simulink model "Ext_Springs_CS9"  (Simulink 8.8)
settings: Solver=ode45  StartTime=0  StopTime=10  FixedStep=0.001  RelTol=1e-3  AbsTol=1e-6
PreLoadFcn:
  | cd Extensions/Simulink/Springs
  | spring_e_class
  | cd ../../..
undefined symbols (not defined in the file): FS_COMP_TABLE_F, FS_COMP_TABLE_R
libraries: Solver_SF x1
settings Model: Creator=dhall  LastModifiedBy=mkhan  ExtModeTrigMode=oneshot  ExtModeArmWhenConnect=off
settings DataIOCC: LimitDataPoints=off  SignalLoggingName=sigsOut
settings OptimizationCC: BooleanDataType=off  ExpressionDepthLimit=2147483647
settings DebuggingCC: SaveWithParameterizedLinksMsg=none  SignalResolutionControl=TryResolveAllWithWarning  MultiTaskDSMMsg=warning  MultiTaskCondExecSysMsg=none  SFExecutionAtInitializationDiag=warning
settings HardwareCC: TargetUnknown=on
settings RTWCC: TemplateMakefile=grt_vc.tmf
settings GRTTargetCC: TargetFcnLib=ansi_tfl_tmw.mat
settings ConfigComp: CovSFcnEnable=off

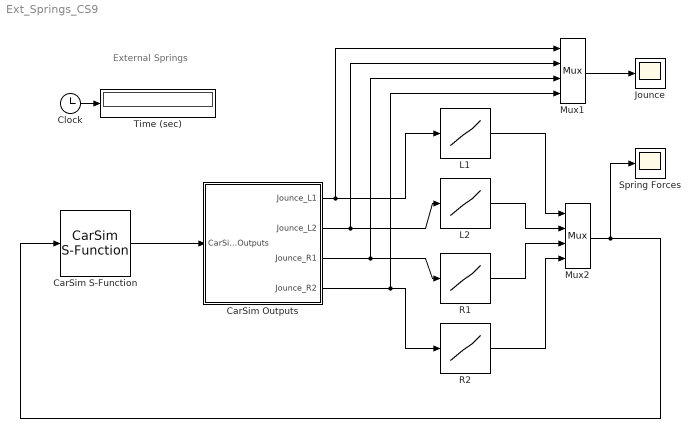
== system Ext_Springs_CS9 ==
  note: External Springs
  CarSim Outputs : Subsystem
  CarSim S-Function : Solver_SF/CarSim S-Function  Priority=1  SIMFILE=simfile.sim  Run_RTs=off  vs_state_ind=Run  StopMode_ind=Vehicle Model
  Clock : Clock
  Jounce : Scope
  L1 : Lookup  InputValues=FS_COMP_TABLE_F(:,1)  Table=FS_COMP_TABLE_F(:,2)  SaturateOnIntegerOverflow=on
  L2 : Lookup  InputValues=FS_COMP_TABLE_R(:,1)  Table=FS_COMP_TABLE_R(:,2)  SaturateOnIntegerOverflow=on
  Mux1 : Mux
  Mux2 : Mux
  R1 : Lookup  InputValues=FS_COMP_TABLE_F(:,1)  Table=FS_COMP_TABLE_F(:,2)  SaturateOnIntegerOverflow=on
  R2 : Lookup  InputValues=FS_COMP_TABLE_R(:,1)  Table=FS_COMP_TABLE_R(:,2)  SaturateOnIntegerOverflow=on
  Spring Forces : Scope
  Time (sec) : Display
      settings: Format=bank  Decimation=100
  wires:
  Mux1/1 -> Jounce/1
  CarSim Outputs/1(Jounce_L1) -> L1/1, Mux1/1
  CarSim Outputs/2(Jounce_L2) -> L2/1, Mux1/2
  CarSim Outputs/3(Jounce_R1) -> R1/1, Mux1/3
  CarSim Outputs/4(Jounce_R2) -> R2/1, Mux1/4
  L1/1 -> Mux2/1
  L2/1 -> Mux2/2
  R1/1 -> Mux2/3
  R2/1 -> Mux2/4
  Clock/1 -> Time (sec)/1
  Mux2/1 -> Spring Forces/1, CarSim S-Function/1
  CarSim S-Function/1 -> CarSim Outputs/1(CarSim Outputs)

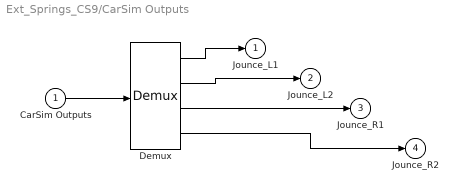
== system Ext_Springs_CS9/CarSim Outputs ==
  CarSim Outputs : Inport
  Demux : Demux
      settings: DisplayOption=none
  Jounce_L1 : Outport  InitialOutput=0
  Jounce_L2 : Outport  Port=2  InitialOutput=0
  Jounce_R1 : Outport  Port=3  InitialOutput=0
  Jounce_R2 : Outport  Port=4  InitialOutput=0
  wires:
  CarSim Outputs/1 -> Demux/1
  Demux/1 -> Jounce_L1/1
  Demux/2 -> Jounce_L2/1
  Demux/3 -> Jounce_R1/1
  Demux/4 -> Jounce_R2/1
